simulink model "pid_tracker"  (R2024a)
settings: Solver=ode23t  StartTime=0.0  StopTime=0.1  MaxStep=1e-5  RelTol=1e-3
libraries: fl_lib x15, ee_lib x15, nesl_utility x14, eePwmGenerator x1, mcbcontrolslib x1, slpidlib x1, simulink x1
settings Model: Creator=SHARISH  LastModifiedBy=SHARI

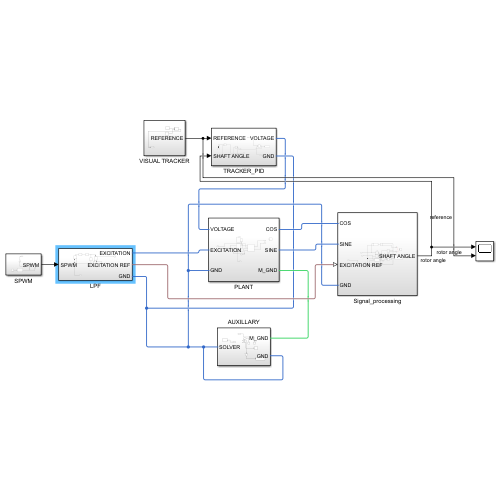
[thumbnail: Simulink's stored preview of the top-level diagram]
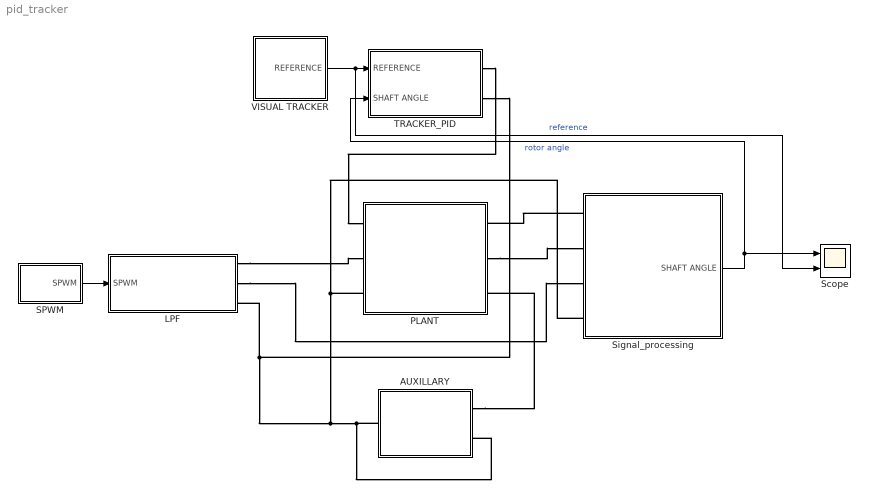
== system pid_tracker ==
  AUXILLARY : Subsystem
  LPF : Subsystem
  PLANT : Subsystem
  SPWM : Subsystem
  Scope : Scope  NumInputPorts=2
  Signal_processing : Subsystem
  TRACKER_PID : Subsystem
  VISUAL TRACKER : Subsystem
  wires:
  SPWM/1(SPWM) -> LPF/1(SPWM)
  Signal_processing/1(SHAFT ANGLE) -> Scope/1, TRACKER_PID/2("SHAFT ANGLE ")  "rotor angle"
  VISUAL TRACKER/1(REFERENCE) -> Scope/2, TRACKER_PID/1("REFERENCE  ")  "reference"
  connections:
  LPF/RConn2 -- Signal_processing/LConn3
  AUXILLARY/LConn2 -- AUXILLARY/RConn1 -- TRACKER_PID/RConn2 -- LPF/RConn3 -- PLANT/LConn3 -- Signal_processing/LConn4
  Signal_processing/LConn1 -- PLANT/RConn1
  PLANT/RConn2 -- Signal_processing/LConn2
  LPF/RConn1 -- PLANT/LConn2
  AUXILLARY/LConn1 -- PLANT/RConn3
  TRACKER_PID/RConn1 -- PLANT/LConn1

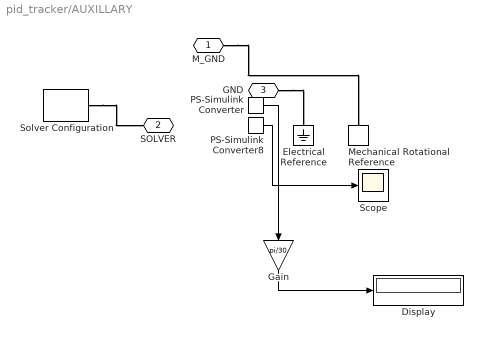
== system pid_tracker/AUXILLARY ==
  Display : Display
  Electrical Reference : fl_lib/Electrical/Electrical Elements/Electrical Reference
  Gain : Gain  Gain=pi/30
  Mechanical Rotational Reference : fl_lib/Mechanical/Rotational Elements/Mechanical Rotational Reference
  PS-Simulink Converter : nesl_utility/PS-Simulink Converter  PhysicalDomain=network_engine_domain  SubClassName=ps_output  LeftPortType=input  RightPortType=output  PseudoPeriodic=off  Frequencies=[]  VectorFormat=inherit  Unit=inherit  AffineConversion=off
  PS-Simulink Converter8 : nesl_utility/PS-Simulink Converter  PhysicalDomain=network_engine_domain  SubClassName=ps_output  LeftPortType=input  RightPortType=output  PseudoPeriodic=off  Frequencies=[]  VectorFormat=inherit  Unit=inherit  AffineConversion=off
  Scope : Scope
  Solver Configuration : nesl_utility/Solver Configuration  PhysicalDomain=network_engine_domain  SubClassName=solver  LeftPortType=input  RightPortType=generic  Tones=[]  Harmonics=[]  SimulateNoise=off  Profile=off  UseLocalSampling=off  EnableSwitchedLinearOptims=on  FrequencyDomain=off  UseCCode=off  RelTol=0.001  AbsTol=0.001  MinStep=1e-09  ToWorkspace=off  RevertToSquareIcSolve=off  NumHomotopyIterations=100  PhasorMode=off  PhasorModeNumHarmonics=1  ConsistencySolver=NEWTON_XTOL_AFTER_FTOL  IndexReductionMethod=DerivativeReplacement  DoDC=off  ResidualTolerance=1e-09  ConsistencyTolSource=GLOBAL  ConsistencyAbsTol=0.001  ConsistencyRelTol=0.001  ConsistencyTolFactor=0.001  UseLocalSolver=off  LocalSolverChoice=NE_BACKWARD_EULER_ADVANCER  ResolveIndetEquations=on  FunctionEvalNumThread=1  LocalSolverSampleTime=0.001  DoFixedCost=off  MaxNonlinIter=3  MaxModeIter=2  ComputeImpulses=off  ImpulseIterations=2  LinearAlgebra=auto  LinearAlgebraNumThread=0  EquationFormulation=NE_TIME_EF  DelaysMemoryBudget=1024  AutomaticFiltering=on  FilteringTimeConstant=0.001  PartitionStorageMethod=AS_NEEDED  PartitionMemoryBudget=1024  PartitionMethod=ROBUST  MultibodyUseLocalSolver=off  MultibodyLocalSolverChoice=ODE1  MultibodyLocalSolverSampleTime=0.001
  M_GND : PMIOPort  Side=Left
  SOLVER : PMIOPort  Port=2  Side=Right
  GND : PMIOPort  Port=3  Side=Left
  wires:
  Gain/1 -> Display/1
  PS-Simulink Converter8/1 -> Scope/1
  PS-Simulink Converter/1 -> Gain/1
  connections:
  GND/RConn1 -- Electrical Reference/LConn1
  M_GND/RConn1 -- Mechanical Rotational Reference/LConn1
  Solver Configuration/RConn1 -- SOLVER/RConn1

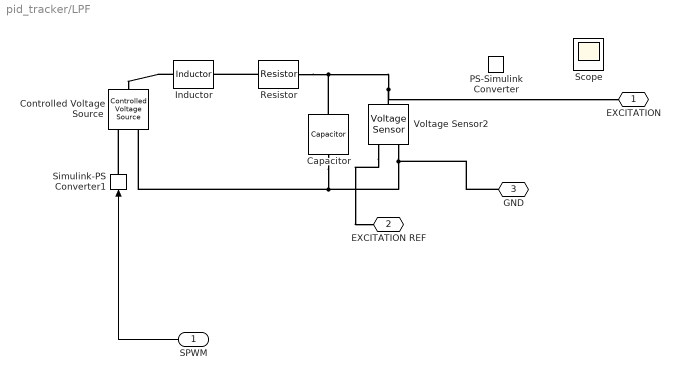
== system pid_tracker/LPF ==
  SPWM : Inport
  Capacitor : fl_lib/Electrical/Electrical Elements/Capacitor  c=1e-6 F  r=1e-6 Ohm  g=0 1/Ohm  i_specify=off  i_priority=None  i=0 A  i_nominal_specify=off  i_nominal_value=1  i_nominal_unit=A  v_specify=off  v_priority=None  v=0 V  v_nominal_specify=off  v_nominal_value=1  v_nominal_unit=V  vc_specify=off  vc_priority=High  vc=0 V  vc_nominal_specify=off  vc_nominal_value=1  vc_nominal_unit=V
  Controlled Voltage Source : fl_lib/Electrical/Electrical Sources/Controlled Voltage Source
  Inductor : ee_lib/Passive/Inductor  l=4.7e-6 H  enable_L_tol=ee.enum.toleranceApplication.none  L_tol=20  tol_distribution=ee.enum.toleranceDistribution.uniform  nSigma=4  r=0 Ohm  g=1e-9 1/Ohm  enable_operating_limits=ee.enum.enable.no  operating_limit_action=ee.enum.passive.reportOpLim.warn  max_working_current=1 A  power_rating=1 W  enable_faults=ee.enum.enable.no  fault_action=simscape.enum.assert.action.none  lambdaPercent=50  k_faulted=0.9999  turnsShort=ee.enum.passive.inductor.turnsShortOption.no  openCct=ee.enum.enable.no  groundShort=ee.enum.passive.inductor.groundShortOption.no  groundShortG=0 1/Ohm  tau_fault=1e-3 s  fault_trigger=ee.enum.faults.faultTrigger.temporal  t_fault=1 s  max_permissible_voltage=100 V  n_fail_on_voltage=1  max_permissible_current=1 A  t_fail_on_current=1 s  i_L_specify=off  i_L_priority=High  i_L=0 A  i_L_nominal_specify=off  i_L_nominal_value=1  i_L_nominal_unit=A  faulted_specify=off  faulted_priority=None  faulted=0
  PS-Simulink Converter : nesl_utility/PS-Simulink Converter  PhysicalDomain=network_engine_domain  SubClassName=ps_output  LeftPortType=input  RightPortType=output  PseudoPeriodic=off  Frequencies=[]  VectorFormat=inherit  Unit=inherit  AffineConversion=off
  Resistor : fl_lib/Electrical/Electrical Elements/Resistor  R=100 Ohm  i_specify=off  i_priority=None  i=0 A  i_nominal_specify=off  i_nominal_value=1  i_nominal_unit=A  v_specify=off  v_priority=None  v=0 V  v_nominal_specify=off  v_nominal_value=1  v_nominal_unit=V
  Scope : Scope
  Simulink-PS Converter1 : nesl_utility/Simulink-PS Converter  PhysicalDomain=network_engine_domain  SubClassName=ps_input  LeftPortType=input  RightPortType=output  PseudoPeriodic=off  Frequencies=[]  NoiseDistribution=none  NoiseParameters=[]  Unit=1  AffineConversion=off  FilteringAndDerivatives=provide  SimscapeFilterOrder=1  InputFilterTimeConstant=0.001  UdotUserProvided=0
  Voltage Sensor2 : fl_lib/Electrical/Electrical Sensors/Voltage Sensor
  EXCITATION : PMIOPort  Side=Right
  EXCITATION REF : PMIOPort  Port=2  Side=Right
  GND : PMIOPort  Port=3  Side=Right
  wires:
  SPWM/1 -> Simulink-PS Converter1/1
  connections:
  Simulink-PS Converter1/RConn1 -- Controlled Voltage Source/RConn1
  Voltage Sensor2/RConn2 -- Capacitor/RConn1 -- Controlled Voltage Source/RConn2 -- GND/RConn1
  Voltage Sensor2/RConn1 -- EXCITATION REF/RConn1
  Voltage Sensor2/LConn1 -- Capacitor/LConn1 -- Resistor/RConn1 -- EXCITATION/RConn1
  Inductor/LConn1 -- Controlled Voltage Source/LConn1
  Resistor/LConn1 -- Inductor/RConn1

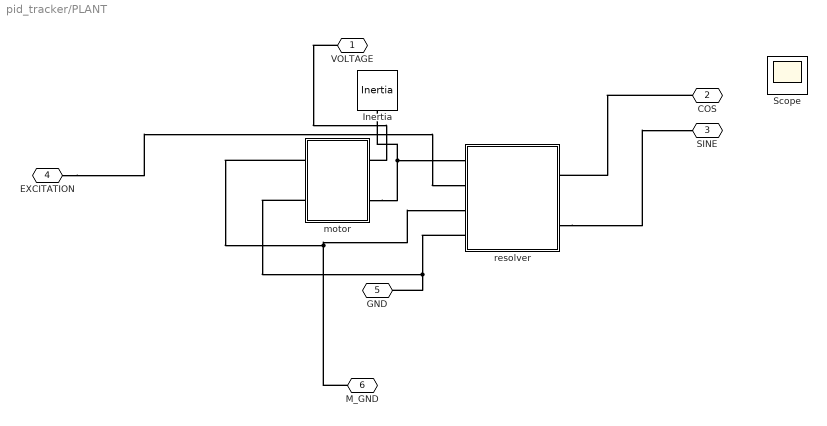
== system pid_tracker/PLANT ==
  Inertia : fl_lib/Mechanical/Rotational Elements/Inertia  inertia=1e-6 kg*m^2  num_ports=foundation.enum.numPorts2.one  w_specify=off  w_priority=High  w=0 rad/s  w_nominal_specify=off  w_nominal_value=1  w_nominal_unit=rad/s  t_specify=off  t_priority=None  t=0 N*m  t_nominal_specify=off  t_nominal_value=1  t_nominal_unit=N*m
  Scope : Scope
  motor : Subsystem
  resolver : Subsystem
  VOLTAGE : PMIOPort  Side=Left
  COS : PMIOPort  Port=2  Side=Right
  SINE : PMIOPort  Port=3  Side=Right
  EXCITATION : PMIOPort  Port=4  Side=Left
  GND : PMIOPort  Port=5  Side=Left
  M_GND : PMIOPort  Port=6  Side=Right
  connections:
  EXCITATION/RConn1 -- resolver/LConn2
  VOLTAGE/RConn1 -- motor/LConn1
  resolver/RConn2 -- SINE/RConn1
  COS/RConn1 -- resolver/RConn1
  Inertia/LConn1 -- motor/LConn2 -- resolver/LConn1
  motor/RConn1 -- resolver/LConn3 -- M_GND/RConn1
  resolver/LConn4 -- GND/RConn1 -- motor/RConn2

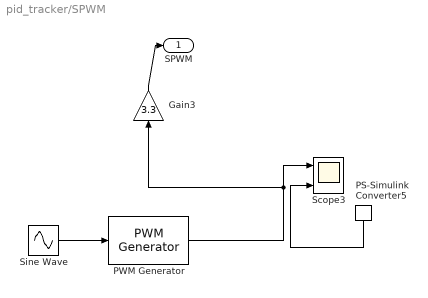
== system pid_tracker/SPWM ==
  Gain3 : Gain  Gain=3.3
  PS-Simulink Converter5 : nesl_utility/PS-Simulink Converter  PhysicalDomain=network_engine_domain  SubClassName=ps_output  LeftPortType=input  RightPortType=output  PseudoPeriodic=off  Frequencies=[]  VectorFormat=inherit  Unit=inherit  AffineConversion=off
  PWM Generator : eePwmGenerator/PWM Generator  CarrCount=Up  Tper=2.8e-5  Tdelay=0  Ts=5e-7
  Scope3 : Scope  NumInputPorts=2
  Sine Wave : Sin  Amplitude=0.5  Bias=0.5  Frequency=2*pi*400  SampleTime=0
  SPWM : Outport
  wires:
  Sine Wave/1 -> PWM Generator/1
  PS-Simulink Converter5/1 -> Scope3/2
  PWM Generator/1 -> Scope3/1, Gain3/1
  Gain3/1 -> SPWM/1

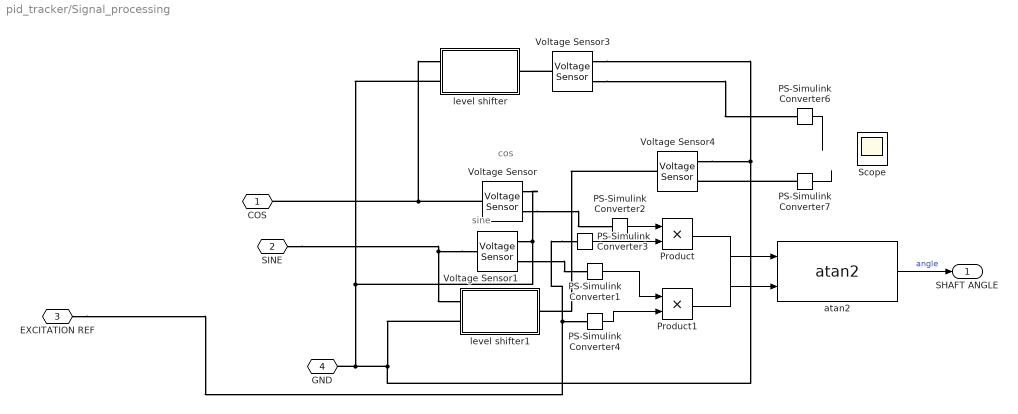
== system pid_tracker/Signal_processing ==
  note: sine
  note: cos
  PS-Simulink Converter{1..4,6..7} (6 alike) : nesl_utility/PS-Simulink Converter  PhysicalDomain=network_engine_domain  SubClassName=ps_output  LeftPortType=input  RightPortType=output  PseudoPeriodic=off  Frequencies=[]  VectorFormat=inherit  Unit=inherit  AffineConversion=off
  Product : Product
  Product1 : Product
  Scope : Scope  NumInputPorts=2
  Voltage Sensor{,1,3..4} (4 alike) : fl_lib/Electrical/Electrical Sensors/Voltage Sensor
  atan2 : mcbcontrolslib/atan2  ApproximationMethod=None  NumberOfIterations=11  NumberOfDataPoints=16  InterpMethod=Flat  outputUnit=Radians  TableDataTypeStr=Inherit: Inherit via input
      settings: LibrarySourceBlock=mcblib/Controls/Math Transforms/atan2
  level shifter : Subsystem
  level shifter1 : Subsystem
  COS : PMIOPort  Side=Left
  SINE : PMIOPort  Port=2  Side=Left
  EXCITATION REF : PMIOPort  Port=3  Side=Left
  GND : PMIOPort  Port=4  Side=Left
  SHAFT ANGLE : Outport
  wires:
  Product1/1 -> atan2/1
  PS-Simulink Converter3/1 -> Product/2
  PS-Simulink Converter4/1 -> Product1/2
  PS-Simulink Converter2/1 -> Product/1
  Product/1 -> atan2/2
  PS-Simulink Converter1/1 -> Product1/1
  atan2/1 -> SHAFT ANGLE/1  "angle"
  PS-Simulink Converter6/1 -> ?
  PS-Simulink Converter7/1 -> ?
  connections:
  Voltage Sensor3/LConn1 -- level shifter/RConn1
  PS-Simulink Converter7/LConn1 -- Voltage Sensor4/RConn1
  PS-Simulink Converter3/LConn1 -- EXCITATION REF/RConn1 -- PS-Simulink Converter4/LConn1
  Voltage Sensor1/LConn1 -- SINE/RConn1 -- level shifter1/LConn1
  Voltage Sensor/RConn2 -- level shifter1/LConn2 -- Voltage Sensor4/RConn2 -- Voltage Sensor3/RConn2 -- GND/RConn1 -- level shifter/LConn2 -- Voltage Sensor1/RConn2
  Voltage Sensor4/LConn1 -- level shifter1/RConn1
  Voltage Sensor3/RConn1 -- PS-Simulink Converter6/LConn1
  Voltage Sensor/RConn1 -- PS-Simulink Converter2/LConn1
  Voltage Sensor1/RConn1 -- PS-Simulink Converter1/LConn1
  Voltage Sensor/LConn1 -- COS/RConn1 -- level shifter/LConn1

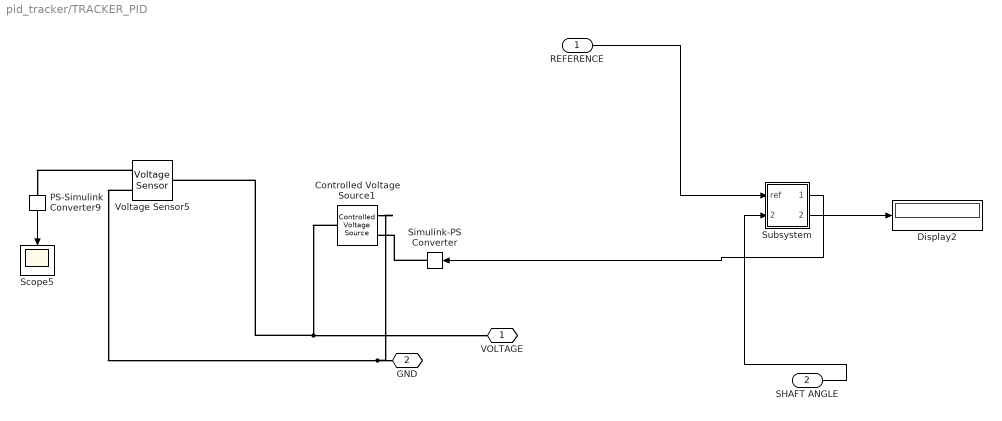
== system pid_tracker/TRACKER_PID ==
  "REFERENCE  " : Inport
  "SHAFT ANGLE " : Inport  Port=2
  Controlled Voltage Source1 : fl_lib/Electrical/Electrical Sources/Controlled Voltage Source
  Display2 : Display
  PS-Simulink Converter9 : nesl_utility/PS-Simulink Converter  PhysicalDomain=network_engine_domain  SubClassName=ps_output  LeftPortType=input  RightPortType=output  PseudoPeriodic=off  Frequencies=[]  VectorFormat=inherit  Unit=inherit  AffineConversion=off
  Scope5 : Scope
  Simulink-PS Converter : nesl_utility/Simulink-PS Converter  PhysicalDomain=network_engine_domain  SubClassName=ps_input  LeftPortType=input  RightPortType=output  PseudoPeriodic=off  Frequencies=[]  NoiseDistribution=none  NoiseParameters=[]  Unit=1  AffineConversion=off  FilteringAndDerivatives=provide  SimscapeFilterOrder=1  InputFilterTimeConstant=0.001  UdotUserProvided=0
  Subsystem : Subsystem
  Voltage Sensor5 : fl_lib/Electrical/Electrical Sensors/Voltage Sensor
  VOLTAGE : PMIOPort  Side=Right
  GND : PMIOPort  Port=2  Side=Right
  wires:
  Subsystem/1(REF) -> Simulink-PS Converter/1
  PS-Simulink Converter9/1 -> Scope5/1
  Subsystem/2(Out2) -> Display2/1
  "SHAFT ANGLE "/1 -> Subsystem/2(angle)
  "REFERENCE  "/1 -> Subsystem/1(ref)
  connections:
  Controlled Voltage Source1/LConn1 -- VOLTAGE/RConn1 -- Voltage Sensor5/LConn1
  Simulink-PS Converter/RConn1 -- Controlled Voltage Source1/RConn1
  Voltage Sensor5/RConn1 -- PS-Simulink Converter9/LConn1
  Voltage Sensor5/RConn2 -- Controlled Voltage Source1/RConn2 -- GND/RConn1

== system pid_tracker/VISUAL TRACKER ==
  Add : Sum
  Sine Wave1 : Sin  Amplitude=0.5  Frequency=2*pi*10  SampleTime=0
  Waveform Generator : simulink/Sources/Waveform Generator  OutMin=[]  OutMax=[]  OutDataTypeStr=double  SelectedSignal=1  Signals=sin(0.3, 10, 0)#  BlockNames=MultiportSwitch_841df5ad9c63433#MultiportSwitch_34cb738a25b4418  SampleTime=0.1
  REFERENCE : Outport
  wires:
  Sine Wave1/1 -> Add/1
  Waveform Generator/1 -> Add/2
  Add/1 -> REFERENCE/1

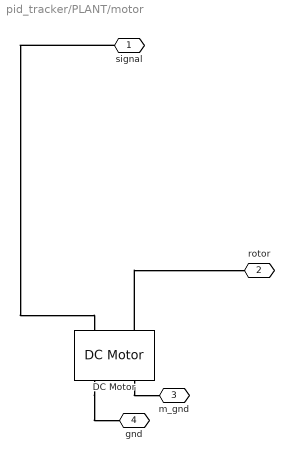
== system pid_tracker/PLANT/motor ==
  DC Motor : ee_lib/Electromechanical/Brushed Motors/DC Motor  field_option=ee.enum.field_option.pm  Rf=100 Ohm  Lf=1 H  Laf=0.15 H  If0=0 A  parameterization=ee.enum.dcparam_option.circuit_param  Ra=5.5 Ohm  La=1.2 mH  emf_or_torque=ee.enum.emf_or_torque.kv  Kv=0.145 V*s/rad  Ki=6.876e-4 N*m/A  T_stall=0.24e-3 N*m  w_max=19100 rpm  w_rated=15000 rpm  P_rated=0.08 W  V_rated=1.5 V  lam_param=ee.enum.lam_param.damping  i_noload=0 A  V_i_noload=1.5 V  J=6.2e-5 kg*m^2  lam=0 N*m*s/rad  speed0=0 rpm  enable_fault_armature=simscape.enum.onoff.off  rev_faulted=1 / 3  G_faulted_armature=1e-5 S  fault_trigger_armature=ee.enum.faults.faultTrigger.temporal  t_fault_armature=1 s  max_permissible_current_armature=inf A  t_fail_on_current_armature=1 s  enable_fault_field=simscape.enum.onoff.off  G_faulted_field=1e-5 S  fault_trigger_field=ee.enum.faults.faultTrigger.temporal  t_fault_field=1 s  max_permissible_current_field=inf A  t_fail_on_current_field=1 s  fault_action=simscape.enum.assert.action.none  alpha=3.93e-3 1/K  Tmeas=25 degC  thermal_mass=100 J/K  initial_temperature=25 degC
  signal : PMIOPort  Side=Left
  rotor : PMIOPort  Port=2  Side=Left
  m_gnd : PMIOPort  Port=3  Side=Right
  gnd : PMIOPort  Port=4  Side=Right
  connections:
  signal/RConn1 -- DC Motor/LConn1
  DC Motor/RConn2 -- m_gnd/RConn1
  DC Motor/RConn1 -- gnd/RConn1
  DC Motor/LConn2 -- rotor/RConn1

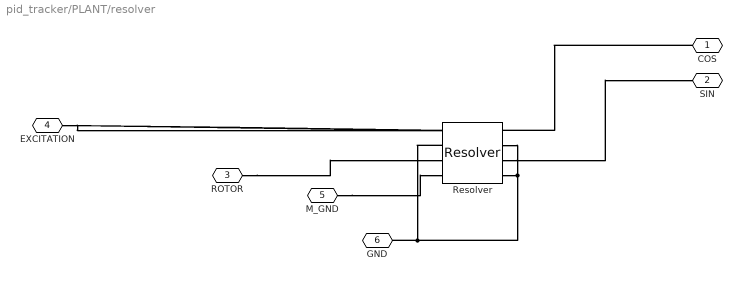
== system pid_tracker/PLANT/resolver ==
  Resolver : ee_lib/Sensors & Transducers/Resolver  parameterization=1  ratio=0.5  Rr=70 Ohm  Rs=180 Ohm  Xr=100 Ohm  Xs=300 Ohm  omega=10 kHz  Lr=0.0016 H  Ls=0.0048 H  k=0.35  N=1  theta_specify=off  theta_priority=None  theta=0 deg  theta_nominal_specify=off  theta_nominal_value=0  theta_nominal_unit=deg
      settings: InternalSimscapePortConfiguration="{\"Bottom\":[],\"Left\":[{\"id\":\"p1\",\"label\":\"p1\",\"type\":\"foundation.electrical.electrical\"},{\"id\":\"p2\",\"label\":\"p2\",\"type\":\"foundation.electrical.electrical\"},{\"id\":\"R\",\"label\":\"R\",\"type\":\"foundation.mechanical.rotational.rotational\"},{\"id\":\"C\",\"label\":\"C\",\"type\":\"foundation.mechanical.rotational.rotational\"}],\"Right\":[{\"id\":\"x1\",\"label\":\"x1\",\"type\":\"foundation.electrical.electrical\"},{\"id\":\"x2\",\"label\":\"x2\",\"type\":\"foundation.electrical.electrical\"},{\"id\":\"y1\",\"label\":\"y1\",\"type\":\"foundation.electrical.electrical\"},{\"id\":\"y2\",\"label\":\"y2\",\"type\":\"foundation.electrical.electrical\"}],\"Top\":[]}"
  COS : PMIOPort  Side=Right
  SIN : PMIOPort  Port=2  Side=Right
  ROTOR : PMIOPort  Port=3  Side=Left
  EXCITATION : PMIOPort  Port=4  Side=Left
  M_GND : PMIOPort  Port=5  Side=Left
  GND : PMIOPort  Port=6  Side=Left
  connections:
  M_GND/RConn1 -- Resolver/LConn4
  Resolver/RConn3 -- SIN/RConn1
  EXCITATION/RConn1 -- Resolver/LConn1
  ROTOR/RConn1 -- Resolver/LConn3
  Resolver/RConn4 -- GND/RConn1 -- Resolver/LConn2 -- Resolver/RConn2
  COS/RConn1 -- Resolver/RConn1

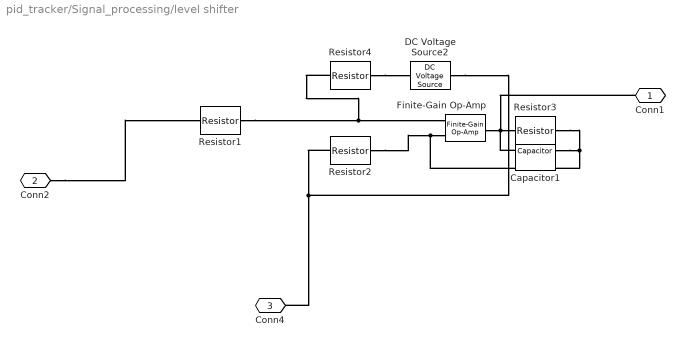
== system pid_tracker/Signal_processing/level shifter ==
  Capacitor1 : fl_lib/Electrical/Electrical Elements/Capacitor  c=1e-9 F  r=1e-6 Ohm  g=0 1/Ohm  i_specify=off  i_priority=None  i=0 A  i_nominal_specify=off  i_nominal_value=1  i_nominal_unit=A  v_specify=off  v_priority=None  v=0 V  v_nominal_specify=off  v_nominal_value=1  v_nominal_unit=V  vc_specify=off  vc_priority=High  vc=0 V  vc_nominal_specify=off  vc_nominal_value=1  vc_nominal_unit=V
  DC Voltage Source2 : ee_lib/Additional Components/SPICE Sources/DC Voltage Source  DC=1.65 V
  Finite-Gain Op-Amp : ee_lib/Integrated Circuits/Finite-Gain Op-Amp  A=1000  Rin=1e6 Ohm  Rout=100 Ohm  Vmin=-15 V  Vmax=15 V  noise_mode=ee.enum.mode.disabled  v_noise=30e-9 V/Hz^(1/2)  noise_prm=ee.enum.ic.noiseParameterization.same  i_noise=0.5e-12 A/Hz^(1/2)  ip_noise=0.5e-12 A/Hz^(1/2)  in_noise=0.5e-12 A/Hz^(1/2)  sample_time=1e-3 s  repeatability=ee.enum.ic.repeatability.notRepeatable  auto_seed_v=1579569999  auto_seed_ip=195013414  auto_seed_in=3162975792  user_seed_v=0  user_seed_ip=0  user_seed_in=0
      settings: InternalSimscapePortConfiguration="{\"Bottom\":[],\"Left\":[{\"id\":\"p\",\"label\":\"+\",\"type\":\"foundation.electrical.electrical\"},{\"id\":\"n\",\"label\":\"-\",\"type\":\"foundation.electrical.electrical\"}],\"Right\":[{\"id\":\"out\",\"label\":\"\",\"type\":\"foundation.electrical.electrical\"}],\"Top\":[]}"
  Resistor1 : ee_lib/Passive/Resistor  R=10 kOhm  enable_R_tol=ee.enum.toleranceApplication.none  R_tol=5  tol_distribution=ee.enum.toleranceDistribution.uniform  nSigma=4  enable_operating_limits=ee.enum.enable.no  operating_limit_action=ee.enum.passive.reportOpLim.warn  power_rating=1 W  max_working_voltage=100 V  enable_faults=ee.enum.enable.no  fault_action=simscape.enum.assert.action.none  R_faulted=inf Ohm  fault_trigger=ee.enum.faults.faultTrigger.temporal  t_fault=1 s  max_permissible_current=1 A  t_fail_on_current=1 s  noise_mode=ee.enum.sources.noise.Disabled  Tdevice=25 degC  sample_time=1e-3 s  repeatability=ee.enum.ic.repeatability.notRepeatable  user_seed=0  auto_seed=1855797429  faulted_specify=off  faulted_priority=None  faulted=0  power_derating_T1=70 degC  power_derating_T2=155 degC  operating_temperature_range_vec=[-50, 150] degC  alpha=3.93e-3 1/K  Tmeas=25 degC  thermal_mass=100 J/K  temperature_specify=off  temperature_priority=High  temperature=298.15 K  temperature_nominal_specify=off  temperature_nominal_value=1  temperature_nominal_unit=K
  Resistor2 : ee_lib/Passive/Resistor  R=10 kOhm  enable_R_tol=ee.enum.toleranceApplication.none  R_tol=5  tol_distribution=ee.enum.toleranceDistribution.uniform  nSigma=4  enable_operating_limits=ee.enum.enable.no  operating_limit_action=ee.enum.passive.reportOpLim.warn  power_rating=1 W  max_working_voltage=100 V  enable_faults=ee.enum.enable.no  fault_action=simscape.enum.assert.action.none  R_faulted=inf Ohm  fault_trigger=ee.enum.faults.faultTrigger.temporal  t_fault=1 s  max_permissible_current=1 A  t_fail_on_current=1 s  noise_mode=ee.enum.sources.noise.Disabled  Tdevice=25 degC  sample_time=1e-3 s  repeatability=ee.enum.ic.repeatability.notRepeatable  user_seed=0  auto_seed=1243900874  faulted_specify=off  faulted_priority=None  faulted=0  power_derating_T1=70 degC  power_derating_T2=155 degC  operating_temperature_range_vec=[-50, 150] degC  alpha=3.93e-3 1/K  Tmeas=25 degC  thermal_mass=100 J/K  temperature_specify=off  temperature_priority=High  temperature=298.15 K  temperature_nominal_specify=off  temperature_nominal_value=1  temperature_nominal_unit=K
  Resistor3 : ee_lib/Passive/Resistor  R=10 kOhm  enable_R_tol=ee.enum.toleranceApplication.none  R_tol=5  tol_distribution=ee.enum.toleranceDistribution.uniform  nSigma=4  enable_operating_limits=ee.enum.enable.no  operating_limit_action=ee.enum.passive.reportOpLim.warn  power_rating=1 W  max_working_voltage=100 V  enable_faults=ee.enum.enable.no  fault_action=simscape.enum.assert.action.none  R_faulted=inf Ohm  fault_trigger=ee.enum.faults.faultTrigger.temporal  t_fault=1 s  max_permissible_current=1 A  t_fail_on_current=1 s  noise_mode=ee.enum.sources.noise.Disabled  Tdevice=25 degC  sample_time=1e-3 s  repeatability=ee.enum.ic.repeatability.notRepeatable  user_seed=0  auto_seed=3117027204  faulted_specify=off  faulted_priority=None  faulted=0  power_derating_T1=70 degC  power_derating_T2=155 degC  operating_temperature_range_vec=[-50, 150] degC  alpha=3.93e-3 1/K  Tmeas=25 degC  thermal_mass=100 J/K  temperature_specify=off  temperature_priority=High  temperature=298.15 K  temperature_nominal_specify=off  temperature_nominal_value=1  temperature_nominal_unit=K
  Resistor4 : ee_lib/Passive/Resistor  R=10 kOhm  enable_R_tol=ee.enum.toleranceApplication.none  R_tol=5  tol_distribution=ee.enum.toleranceDistribution.uniform  nSigma=4  enable_operating_limits=ee.enum.enable.no  operating_limit_action=ee.enum.passive.reportOpLim.warn  power_rating=1 W  max_working_voltage=100 V  enable_faults=ee.enum.enable.no  fault_action=simscape.enum.assert.action.none  R_faulted=inf Ohm  fault_trigger=ee.enum.faults.faultTrigger.temporal  t_fault=1 s  max_permissible_current=1 A  t_fail_on_current=1 s  noise_mode=ee.enum.sources.noise.Disabled  Tdevice=25 degC  sample_time=1e-3 s  repeatability=ee.enum.ic.repeatability.notRepeatable  user_seed=0  auto_seed=834788543  faulted_specify=off  faulted_priority=None  faulted=0  power_derating_T1=70 degC  power_derating_T2=155 degC  operating_temperature_range_vec=[-50, 150] degC  alpha=3.93e-3 1/K  Tmeas=25 degC  thermal_mass=100 J/K  temperature_specify=off  temperature_priority=High  temperature=298.15 K  temperature_nominal_specify=off  temperature_nominal_value=1  temperature_nominal_unit=K
  Conn1 : PMIOPort  Side=Right
  Conn2 : PMIOPort  Port=2  Side=Left
  Conn4 : PMIOPort  Port=3  Side=Left
  connections:
  Resistor2/RConn1 -- Finite-Gain Op-Amp/LConn2 -- Resistor3/RConn1 -- Capacitor1/RConn1
  Conn2/RConn1 -- Resistor1/LConn1
  Finite-Gain Op-Amp/RConn1 -- Resistor3/LConn1 -- Capacitor1/LConn1 -- Conn1/RConn1
  Resistor4/RConn1 -- DC Voltage Source2/LConn1
  Resistor4/LConn1 -- Finite-Gain Op-Amp/LConn1 -- Resistor1/RConn1
  Resistor2/LConn1 -- Conn4/RConn1 -- DC Voltage Source2/RConn1

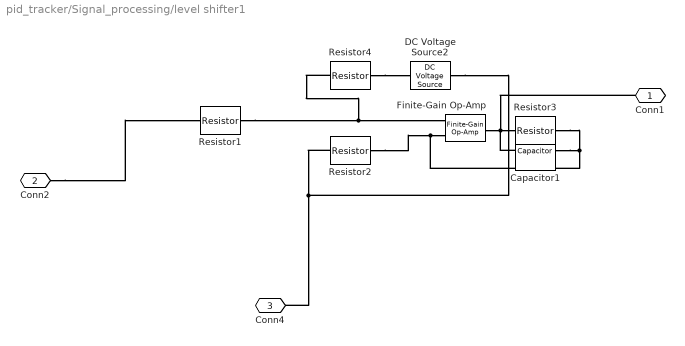
== system pid_tracker/Signal_processing/level shifter1 ==
  Capacitor1 : fl_lib/Electrical/Electrical Elements/Capacitor  c=1e-9 F  r=1e-6 Ohm  g=0 1/Ohm  i_specify=off  i_priority=None  i=0 A  i_nominal_specify=off  i_nominal_value=1  i_nominal_unit=A  v_specify=off  v_priority=None  v=0 V  v_nominal_specify=off  v_nominal_value=1  v_nominal_unit=V  vc_specify=off  vc_priority=High  vc=0 V  vc_nominal_specify=off  vc_nominal_value=1  vc_nominal_unit=V
  DC Voltage Source2 : ee_lib/Additional Components/SPICE Sources/DC Voltage Source  DC=1.65 V
  Finite-Gain Op-Amp : ee_lib/Integrated Circuits/Finite-Gain Op-Amp  A=1000  Rin=1e6 Ohm  Rout=100 Ohm  Vmin=-15 V  Vmax=15 V  noise_mode=ee.enum.mode.disabled  v_noise=30e-9 V/Hz^(1/2)  noise_prm=ee.enum.ic.noiseParameterization.same  i_noise=0.5e-12 A/Hz^(1/2)  ip_noise=0.5e-12 A/Hz^(1/2)  in_noise=0.5e-12 A/Hz^(1/2)  sample_time=1e-3 s  repeatability=ee.enum.ic.repeatability.notRepeatable  auto_seed_v=2948897582  auto_seed_ip=221036891  auto_seed_in=3508195287  user_seed_v=0  user_seed_ip=0  user_seed_in=0
      settings: InternalSimscapePortConfiguration="{\"Bottom\":[],\"Left\":[{\"id\":\"p\",\"label\":\"+\",\"type\":\"foundation.electrical.electrical\"},{\"id\":\"n\",\"label\":\"-\",\"type\":\"foundation.electrical.electrical\"}],\"Right\":[{\"id\":\"out\",\"label\":\"\",\"type\":\"foundation.electrical.electrical\"}],\"Top\":[]}"
  Resistor1 : ee_lib/Passive/Resistor  R=10 kOhm  enable_R_tol=ee.enum.toleranceApplication.none  R_tol=5  tol_distribution=ee.enum.toleranceDistribution.uniform  nSigma=4  enable_operating_limits=ee.enum.enable.no  operating_limit_action=ee.enum.passive.reportOpLim.warn  power_rating=1 W  max_working_voltage=100 V  enable_faults=ee.enum.enable.no  fault_action=simscape.enum.assert.action.none  R_faulted=inf Ohm  fault_trigger=ee.enum.faults.faultTrigger.temporal  t_fault=1 s  max_permissible_current=1 A  t_fail_on_current=1 s  noise_mode=ee.enum.sources.noise.Disabled  Tdevice=25 degC  sample_time=1e-3 s  repeatability=ee.enum.ic.repeatability.notRepeatable  user_seed=0  auto_seed=1628565735  faulted_specify=off  faulted_priority=None  faulted=0  power_derating_T1=70 degC  power_derating_T2=155 degC  operating_temperature_range_vec=[-50, 150] degC  alpha=3.93e-3 1/K  Tmeas=25 degC  thermal_mass=100 J/K  temperature_specify=off  temperature_priority=High  temperature=298.15 K  temperature_nominal_specify=off  temperature_nominal_value=1  temperature_nominal_unit=K
  Resistor2 : ee_lib/Passive/Resistor  R=10 kOhm  enable_R_tol=ee.enum.toleranceApplication.none  R_tol=5  tol_distribution=ee.enum.toleranceDistribution.uniform  nSigma=4  enable_operating_limits=ee.enum.enable.no  operating_limit_action=ee.enum.passive.reportOpLim.warn  power_rating=1 W  max_working_voltage=100 V  enable_faults=ee.enum.enable.no  fault_action=simscape.enum.assert.action.none  R_faulted=inf Ohm  fault_trigger=ee.enum.faults.faultTrigger.temporal  t_fault=1 s  max_permissible_current=1 A  t_fail_on_current=1 s  noise_mode=ee.enum.sources.noise.Disabled  Tdevice=25 degC  sample_time=1e-3 s  repeatability=ee.enum.ic.repeatability.notRepeatable  user_seed=0  auto_seed=3669867250  faulted_specify=off  faulted_priority=None  faulted=0  power_derating_T1=70 degC  power_derating_T2=155 degC  operating_temperature_range_vec=[-50, 150] degC  alpha=3.93e-3 1/K  Tmeas=25 degC  thermal_mass=100 J/K  temperature_specify=off  temperature_priority=High  temperature=298.15 K  temperature_nominal_specify=off  temperature_nominal_value=1  temperature_nominal_unit=K
  Resistor3 : ee_lib/Passive/Resistor  R=10 kOhm  enable_R_tol=ee.enum.toleranceApplication.none  R_tol=5  tol_distribution=ee.enum.toleranceDistribution.uniform  nSigma=4  enable_operating_limits=ee.enum.enable.no  operating_limit_action=ee.enum.passive.reportOpLim.warn  power_rating=1 W  max_working_voltage=100 V  enable_faults=ee.enum.enable.no  fault_action=simscape.enum.assert.action.none  R_faulted=inf Ohm  fault_trigger=ee.enum.faults.faultTrigger.temporal  t_fault=1 s  max_permissible_current=1 A  t_fail_on_current=1 s  noise_mode=ee.enum.sources.noise.Disabled  Tdevice=25 degC  sample_time=1e-3 s  repeatability=ee.enum.ic.repeatability.notRepeatable  user_seed=0  auto_seed=1003685772  faulted_specify=off  faulted_priority=None  faulted=0  power_derating_T1=70 degC  power_derating_T2=155 degC  operating_temperature_range_vec=[-50, 150] degC  alpha=3.93e-3 1/K  Tmeas=25 degC  thermal_mass=100 J/K  temperature_specify=off  temperature_priority=High  temperature=298.15 K  temperature_nominal_specify=off  temperature_nominal_value=1  temperature_nominal_unit=K
  Resistor4 : ee_lib/Passive/Resistor  R=10 kOhm  enable_R_tol=ee.enum.toleranceApplication.none  R_tol=5  tol_distribution=ee.enum.toleranceDistribution.uniform  nSigma=4  enable_operating_limits=ee.enum.enable.no  operating_limit_action=ee.enum.passive.reportOpLim.warn  power_rating=1 W  max_working_voltage=100 V  enable_faults=ee.enum.enable.no  fault_action=simscape.enum.assert.action.none  R_faulted=inf Ohm  fault_trigger=ee.enum.faults.faultTrigger.temporal  t_fault=1 s  max_permissible_current=1 A  t_fail_on_current=1 s  noise_mode=ee.enum.sources.noise.Disabled  Tdevice=25 degC  sample_time=1e-3 s  repeatability=ee.enum.ic.repeatability.notRepeatable  user_seed=0  auto_seed=2304370027  faulted_specify=off  faulted_priority=None  faulted=0  power_derating_T1=70 degC  power_derating_T2=155 degC  operating_temperature_range_vec=[-50, 150] degC  alpha=3.93e-3 1/K  Tmeas=25 degC  thermal_mass=100 J/K  temperature_specify=off  temperature_priority=High  temperature=298.15 K  temperature_nominal_specify=off  temperature_nominal_value=1  temperature_nominal_unit=K
  Conn1 : PMIOPort  Side=Right
  Conn2 : PMIOPort  Port=2  Side=Left
  Conn4 : PMIOPort  Port=3  Side=Left
  connections:
  Resistor2/RConn1 -- Finite-Gain Op-Amp/LConn2 -- Resistor3/RConn1 -- Capacitor1/RConn1
  Conn2/RConn1 -- Resistor1/LConn1
  Finite-Gain Op-Amp/RConn1 -- Resistor3/LConn1 -- Capacitor1/LConn1 -- Conn1/RConn1
  Resistor4/RConn1 -- DC Voltage Source2/LConn1
  Resistor4/LConn1 -- Finite-Gain Op-Amp/LConn1 -- Resistor1/RConn1
  Resistor2/LConn1 -- Conn4/RConn1 -- DC Voltage Source2/RConn1

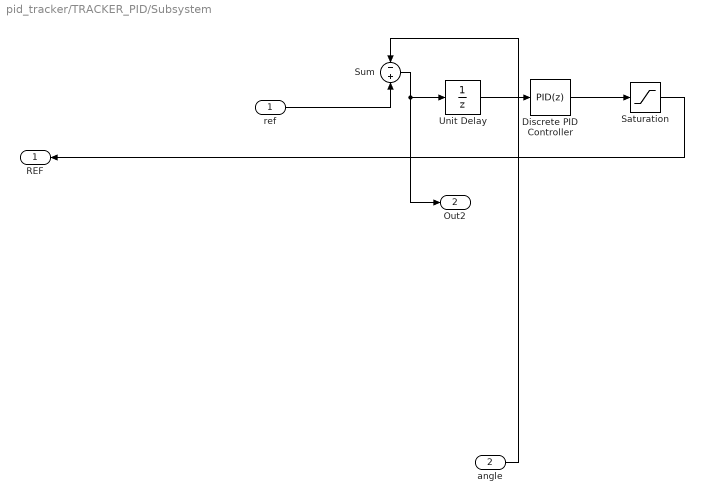
== system pid_tracker/TRACKER_PID/Subsystem ==
  ref : Inport
  angle : Inport  Port=2
  Discrete PID Controller : slpidlib/PID Controller  Controller=PID  Form=Parallel  TimeDomain=Discrete-time  UseExternalTs=off  SampleTime=0.2e-3  IntegratorMethod=Forward Euler  FilterMethod=Forward Euler  ControllerParametersSource=internal  P=9  I=1  UseKiTs=off  D=30  UseExternalDerivativeSource=off  N=100  UseFilter=on  TunerSelectOption=Transfer Function Based (PID Tuner App)  InitialConditionSource=internal  InitialConditionForIntegrator=0  InitialConditionForFilter=0  DifferentiatorICPrevScaledInput=0  ExternalReset=none  TrackingMode=off  Kt=1  LimitOutput=on  SatLimitsSource=internal  UpperSaturationLimit=12  LowerSaturationLimit=-12  LinearizeAsGain=off  AntiWindupMode=none  Kb=1  LimitIntegrator=off  UpperIntegratorSaturationLimit=inf  LowerIntegratorSaturationLimit=-inf  POutMin=[]  POutMax=[]  IOutMin=[]  IOutMax=[]  DOutMin=[]  DOutMax=[]  NOutMin=[]  NOutMax=[]  SumOutMin=[]  SumOutMax=[]  SaturationOutMin=[]  SaturationOutMax=[]  PParamMin=[]  PParamMax=[]  IParamMin=[]  IParamMax=[]  DParamMin=[]  DParamMax=[]  NParamMin=[]  NParamMax=[]  KbParamMin=[]  KbParamMax=[]  KtParamMin=[]  KtParamMax=[]  KbOutMin=[]  KbOutMax=[]  KtOutMin=[]  KtOutMax=[]  IntegratorOutMin=[]  IntegratorOutMax=[]  FilterOutMin=[]  FilterOutMax=[]  SumI1OutMin=[]  SumI1OutMax=[]  SumI2OutMin=[]  SumI2OutMax=[]  SumI3OutMin=[]  SumI3OutMax=[]  SumI4OutMin=[]  SumI4OutMax=[]  SumDOutMin=[]  SumDOutMax=[]  DifferentiatorOutMin=[]  DifferentiatorOutMax=[]  FilterDiffOutCoefMin=[]  FilterDiffOutCoefMax=[]  ReciprocalOutMin=[]  ReciprocalOutMax=[]  SumDenOutMin=[]  SumDenOutMax=[]  SumNumOutMin=[]  SumNumOutMax=[]  DivideOutMin=[]  DivideOutMax=[]  UdiffTsProdOutMin=[]  UdiffTsProdOutMax=[]  NTsProdOutMin=[]  NTsProdOutMax=[]  UintegralTsProdOutMin=[]  UintegralTsProdOutMax=[]  UngainTsProdOutMin=[]  UngainTsProdOutMax=[]  ClampingZeroOutDataTypeStr=Inherit: Inherit via back propagation  ClampingZeroOutMin=[]  ClampingZeroOutMax=[]  FilterDenConstantOutDataTypeStr=Inherit: Inherit via back propagation  FilterDenConstantOutMin=[]  FilterDenConstantOutMax=[]  PCopyOutDataTypeStr=Inherit: Inherit via back propagation  PCopyOutMin=[]  PCopyOutMax=[]  NCopyOutDataTypeStr=Inherit: Inherit via back propagation  NCopyOutMin=[]  NCopyOutMax=[]  IntegratorContinuousStateAttributes=''  IntegratorStateMustResolveToSignalObject=off  IntegratorRTWStateStorageClass=Auto  FilterContinuousStateAttributes=''  FilterStateMustResolveToSignalObject=off  FilterRTWStateStorageClass=Auto  ParallelPVariant=InternalParameters  IdealPVariant=Disabled  IVariant=InternalParameters  DVariant=InternalParameters  IntegratorVariant=Discrete  SatVariant=Enabled  AWVariant=Passthrough  PCopyVariant=Disabled  TRVariant=Disabled  FdbkBlocksVariant=Forward  IdealPFdbkVariant=Disabled  SatFdbkVariant=Disabled  DerivativeFilterVariant=ForwardEulerFilter  NVariant=InternalParameters  NCopyVariant=Disabled  FilterICVariant=InternalICsFilter  IntegratorICVariant=InternalICs  ExternalResetVariant=Disabled  TRSumVariant=Passthrough  SumFdbkVariant=Disabled  SumVariant=Sum_PID  TsampFilterVariant=InternalTs  TsampNgainVariant=Passthrough  TsampIntegralVariant=Disabled_SignalSpec  ExternalSaturationOutDataTypeStr=Inherit: Same as second input  DerivativeSourceVariant=ErrorSignal
      settings: LibrarySourceBlock=simulink/Discrete/Discrete PID Controller
  Saturation : Saturate  UpperLimit=12  LowerLimit=-12
  Sum : Sum  Inputs=-+
  Unit Delay : UnitDelay  SampleTime=-1  HasFrameUpgradeWarning=on
  REF : Outport
  Out2 : Outport  Port=2
  wires:
  ref/1 -> Sum/2
  Sum/1 -> Out2/1, Unit Delay/1
  Unit Delay/1 -> Discrete PID Controller/1
  Discrete PID Controller/1 -> Saturation/1
  Saturation/1 -> REF/1
  angle/1 -> Sum/1
